simulink model "DC_SIM"  (R2016b)
settings: Solver=ode2  StartTime=0.0  StopTime=10  FixedStep=1e-2  RelTol=1e-3
values from neighbouring files (symbols this model uses):
  D = b_hole(3)    [PSO_update_DC.m]    (also in test_function.m = a(3,1))
  I = b_hole(2)    [PSO_update_DC.m]    (also in test_function.m = a(2,1))
  P = b_hole(1)    [PSO_update_DC.m]    (also in test_function.m = a(1,1))
libraries: simulink x1
settings Model: Creator=tiend  LastModifiedBy=tiend

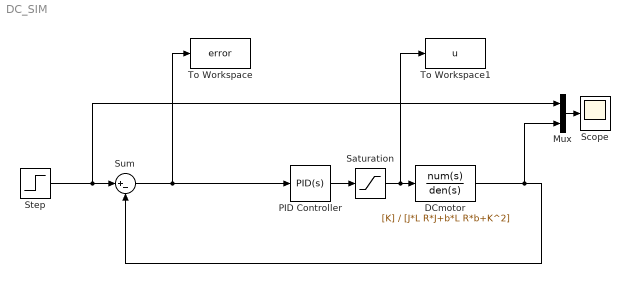
== system DC_SIM ==
  DCmotor : TransferFcn  Numerator=[K]  Denominator=[J*L R*J+b*L R*b+K^2]  mask{K=0.01, J=0.01, b=0.1, L=0.5, R=1}
  Mux : Mux  Inputs=2
  PID Controller : simulink/Continuous/PID Controller  Controller=PID  TimeDomain=Continuous-time  SampleTime=-1  IntegratorMethod=Forward Euler  FilterMethod=Forward Euler  Form=Parallel  UseFilter=on  ControllerParametersSource=internal  P=P  I=I  D=D  N=100  InitialConditionSource=internal  InitialConditionForIntegrator=0  InitialConditionForFilter=0  ExternalReset=none  LimitOutput=off  UpperSaturationLimit=inf  LowerSaturationLimit=-inf  LinearizeAsGain=on  AntiWindupMode=none  Kb=1  TrackingMode=off  Kt=1  PParamMin=[]  PParamMax=[]  IParamMin=[]  IParamMax=[]  DParamMin=[]  DParamMax=[]  NParamMin=[]  NParamMax=[]  KbParamMin=[]  KbParamMax=[]  KtParamMin=[]  KtParamMax=[]  POutMin=[-512]  POutMax=[512]  IOutMin=[-512]  IOutMax=[512]  DOutMin=[-512]  DOutMax=[512]  NOutMin=[]  NOutMax=[]  KbOutMin=[]  KbOutMax=[]  KtOutMin=[]  KtOutMax=[]  IntegratorOutMin=[]  IntegratorOutMax=[]  FilterOutMin=[]  FilterOutMax=[]  SumOutMin=[]  SumOutMax=[]  SumI1OutMin=[]  SumI1OutMax=[]  SumI2OutMin=[]  SumI2OutMax=[]  SumI3OutMin=[]  SumI3OutMax=[]  SumDOutMin=[]  SumDOutMax=[]  SaturationOutMin=[]  SaturationOutMax=[]  IntegratorContinuousStateAttributes=''  IntegratorStateMustResolveToSignalObject=off  IntegratorRTWStateStorageClass=Auto  FilterContinuousStateAttributes=''  FilterStateMustResolveToSignalObject=off  FilterRTWStateStorageClass=Auto  DifferentiatorICPrevScaledInput=0  DifferentiatorOutMin=[]  DifferentiatorOutMax=[]
  Saturation : Saturate  UpperLimit=500  LowerLimit=-500
  Scope : Scope
  Step : Step  Time=0.2  After=10  SampleTime=0
  Sum : Sum  Inputs=|+-
  To Workspace : ToWorkspace  VariableName=error  SampleTime=-1
  To Workspace1 : ToWorkspace  VariableName=u  SampleTime=-1
  wires:
  Sum/1 -> PID Controller/1, To Workspace/1
  DCmotor/1 -> Mux/2, Sum/2
  PID Controller/1 -> Saturation/1
  Mux/1 -> Scope/1
  Step/1 -> Mux/1, Sum/1
  Saturation/1 -> To Workspace1/1, DCmotor/1
